simulink model "MPC_MG_raw_ver1"  (R2021b)
settings: Solver=ode23tb  StartTime=0.0  StopTime=1  RelTol=1e-3
model workspace (MAT data in the model file):
  Ts = Simulink.Parameter
  Ts.Value = 5e-06
  Ts.DataType = 'auto'
  Ts.Complexity = 'real'
  Ts.Dimensions = [1 1]
  secondary_on = Simulink.Parameter
  secondary_on.DataType = 'auto'
  secondary_on.Complexity = 'real'
  secondary_on.Dimensions = [0 0]
values from neighbouring files (symbols this model uses):
  A = zeros(4,4)    [MPC_MG_script_raw_dmpc.m]    (also in MPG_MG_July.m = [0 1 1 1; 1 0 0 0; 1 0 0 0; 1 0 0 0]; MPG_MG_freq_script.m = ones(4) - eye(4); Script.m = [0 1 1 1 ; 1 0 1 1 ; 1 1 0 1 ; 1 1 1 0])
  a12 = 0    [Four_DG_MG_PrimaryOnlyScript.m]    (also in MPC_MG_script_raw_dmpc.m; MPC_MG_secondary_script.m)
  a14 = 0    [Four_DG_MG_PrimaryOnlyScript.m]    (also in MPC_MG_script_raw_dmpc.m; MPC_MG_secondary_script.m)
  a21 = 1    [Four_DG_MG_PrimaryOnlyScript.m]    (also in MPC_MG_script_raw_dmpc.m; MPC_MG_secondary_script.m)
  a23 = 0    [Four_DG_MG_PrimaryOnlyScript.m]    (also in MPC_MG_script_raw_dmpc.m; MPC_MG_secondary_script.m)
  a32 = 1    [Four_DG_MG_PrimaryOnlyScript.m]    (also in MPC_MG_script_raw_dmpc.m; MPC_MG_secondary_script.m)
  a34 = 0    [Four_DG_MG_PrimaryOnlyScript.m]    (also in MPC_MG_script_raw_dmpc.m; MPC_MG_secondary_script.m)
  a41 = 1    [Four_DG_MG_PrimaryOnlyScript.m]    (also in MPC_MG_script_raw_dmpc.m; MPC_MG_secondary_script.m)
  a43 = 0    [Four_DG_MG_PrimaryOnlyScript.m]    (also in MPC_MG_script_raw_dmpc.m; MPC_MG_secondary_script.m)
  b1v = 1    [Four_DG_MG_PrimaryOnlyScript.m]    (also in MPC_MG_script_raw_dmpc.m; MPC_MG_secondary_script.m; MPG_MG_July.m; MPG_MG_freq_script.m)
  b1w = 1    [Four_DG_MG_PrimaryOnlyScript.m]    (also in MPC_MG_script_raw_dmpc.m; MPC_MG_secondary_script.m; MPG_MG_July.m; MPG_MG_freq_script.m)
  b2v = 0    [Four_DG_MG_PrimaryOnlyScript.m]    (also in MPC_MG_script_raw_dmpc.m; MPC_MG_secondary_script.m; MPG_MG_July.m; MPG_MG_freq_script.m)
  b2w = 0    [Four_DG_MG_PrimaryOnlyScript.m]    (also in MPC_MG_script_raw_dmpc.m; MPC_MG_secondary_script.m; MPG_MG_July.m; MPG_MG_freq_script.m)
  b3v = 0    [Four_DG_MG_PrimaryOnlyScript.m]    (also in MPC_MG_script_raw_dmpc.m; MPC_MG_secondary_script.m; MPG_MG_July.m; MPG_MG_freq_script.m)
  b3w = 0    [Four_DG_MG_PrimaryOnlyScript.m]    (also in MPC_MG_script_raw_dmpc.m; MPC_MG_secondary_script.m; MPG_MG_July.m; MPG_MG_freq_script.m)
  b4v = 0    [Four_DG_MG_PrimaryOnlyScript.m]    (also in MPC_MG_script_raw_dmpc.m; MPC_MG_secondary_script.m; MPG_MG_July.m; MPG_MG_freq_script.m)
  b4w = 0    [Four_DG_MG_PrimaryOnlyScript.m]    (also in MPC_MG_script_raw_dmpc.m; MPC_MG_secondary_script.m; MPG_MG_July.m; MPG_MG_freq_script.m)
  C_f = 50e-6    (= 5e-05)    [Four_DG_MG_PrimaryOnlyScript.m]    (also in MPC_MG_script.m; MPC_MG_script_raw_dmpc.m; MPC_MG_secondary_script.m; MPG_MG_July.m)
  cf = 60    [Four_DG_MG_PrimaryOnlyScript.m]    (also in MPC_MG_script_raw_dmpc.m = 40; MPC_MG_secondary_script.m = 40; MPG_MG_July.m = 100; MPG_MG_freq_script.m = 100)
  cv = 60    [Four_DG_MG_PrimaryOnlyScript.m]    (also in MPC_MG_script_raw_dmpc.m = 40; MPC_MG_secondary_script.m = 40; MPG_MG_July.m = 100; MPG_MG_freq_script.m = 100)
  f_c = 5000    [Four_DG_MG_PrimaryOnlyScript.m]    (also in MPC_MG_script.m = 40000; MPC_MG_script_raw_dmpc.m = 40000; MPC_MG_secondary_script.m = 40000; MPG_MG_July.m = 50000)
  kL = 1e-5    (= 1e-05)    [Four_DG_MG_PrimaryOnlyScript.m]    (also in MPC_MG_script.m = 1e-08; MPC_MG_script_raw_dmpc.m = 1e-08; MPC_MG_secondary_script.m = 1e-07; MPG_MG_July.m = 1e-07)
  L_f = 1.35e-3    (= 0.00135)    [Four_DG_MG_PrimaryOnlyScript.m]    (also in MPC_MG_script.m; MPC_MG_script_raw_dmpc.m; MPC_MG_secondary_script.m; MPG_MG_July.m)
  L_in1 = 0.35e-3    (= 0.00035)    [Four_DG_MG_PrimaryOnlyScript.m]    (also in MPC_MG_script.m; MPC_MG_script_raw_dmpc.m; MPC_MG_secondary_script.m; MPG_MG_July.m)
  L_in2 = 0.35e-3    (= 0.00035)    [Four_DG_MG_PrimaryOnlyScript.m]    (also in MPC_MG_script.m; MPC_MG_script_raw_dmpc.m; MPC_MG_secondary_script.m; MPG_MG_July.m)
  L_in3 = 0.35e-3    (= 0.00035)    [Four_DG_MG_PrimaryOnlyScript.m]    (also in MPC_MG_script.m; MPC_MG_script_raw_dmpc.m; MPC_MG_secondary_script.m; MPG_MG_July.m)
  lambda1 = [30000 50000 90000 50000]'    [MPC_MG_script_raw_dmpc.m]    (also in MPG_MG_July.m = [4 4 4 4]'; MPG_MG_freq_script.m = [3 3 3 3]'; Script.m = [1 1 1 1]')
  lambda2 = [5 6 7 6]'    [MPC_MG_script_raw_dmpc.m]    (also in MPG_MG_July.m = [0.5e-2 0.5e-2 0.5e-2 0.5e-2]'; MPG_MG_freq_script.m = [1.1 1.9 1.5 1.2]'; Script.m = [0.8e-2 0.8e-2 0.8e-2 0.8e-2]')
  lambda3 = [80000 80000 900000 80000]'    [MPC_MG_script_raw_dmpc.m]    (also in MPG_MG_July.m = [1e-3 1e-3 1e-3 1e-3]'; MPG_MG_freq_script.m = [9e-4 1.2e-2 3e-3 3e-3]'; Script.m = [1.5e-3 1.5e-3 1.5e-3 1.5e-3]')
  lambda4 = [5000 5000 5000 5000]'    [MPC_MG_script_raw_dmpc.m]
  lambda5 = [150 130 200 130]'    [MPC_MG_script_raw_dmpc.m]
  lambda6 = [5000 2000 1000 2000]'    [MPC_MG_script_raw_dmpc.m]
  LD_ref1 = 800e-6    (= 0.0008)    [Four_DG_MG_PrimaryOnlyScript.m]    (also in MPC_MG_script.m = 0.0003; MPC_MG_script_raw_dmpc.m = 0.0003; MPC_MG_secondary_script.m = 0.0001; MPG_MG_July.m = 0.0004)
  lo_co = 0.2    [Four_DG_MG_PrimaryOnlyScript.m]    (also in MPC_MG_script.m = 0.05; MPC_MG_script_raw_dmpc.m = 0.1; MPC_MG_secondary_script.m = 0.08; MPG_MG_July.m = 0.15)
  m_p1 = 9.4e-5/droopDivide    (= 9.4e-05)    [Four_DG_MG_PrimaryOnlyScript.m]    (also in MPC_MG_script.m; MPC_MG_script_raw_dmpc.m; MPC_MG_secondary_script.m; MPG_MG_July.m)
  m_p2 = 9.4e-5/droopDivide    (= 9.4e-05)    [Four_DG_MG_PrimaryOnlyScript.m]    (also in MPC_MG_script.m; MPC_MG_script_raw_dmpc.m; MPC_MG_secondary_script.m; MPG_MG_July.m)
  m_p3 = 12.5e-5/droopDivide    (= 0.000125)    [Four_DG_MG_PrimaryOnlyScript.m]    (also in MPC_MG_script.m; MPC_MG_script_raw_dmpc.m; MPC_MG_secondary_script.m; MPG_MG_July.m)
  m_p4 = 12.5e-5/droopDivide    (= 0.000125)    [Four_DG_MG_PrimaryOnlyScript.m]    (also in MPC_MG_script.m; MPC_MG_script_raw_dmpc.m; MPC_MG_secondary_script.m; MPG_MG_July.m)
  n_q1 = 1.3e-3/droopDivide2    (= 0.00013)    [Four_DG_MG_PrimaryOnlyScript.m]    (also in MPC_MG_script.m; MPC_MG_script_raw_dmpc.m; MPC_MG_secondary_script.m; MPG_MG_July.m)
  n_q2 = 1.3e-3/droopDivide2    (= 0.00013)    [Four_DG_MG_PrimaryOnlyScript.m]    (also in MPC_MG_script.m; MPC_MG_script_raw_dmpc.m; MPC_MG_secondary_script.m; MPG_MG_July.m)
  n_q3 = 1.5e-3/droopDivide2    (= 0.00015)    [Four_DG_MG_PrimaryOnlyScript.m]    (also in MPC_MG_script.m; MPC_MG_script_raw_dmpc.m; MPC_MG_secondary_script.m; MPG_MG_July.m)
  n_q4 = 1.5e-3/droopDivide2    (= 0.00015)    [Four_DG_MG_PrimaryOnlyScript.m]    (also in MPC_MG_script.m; MPC_MG_script_raw_dmpc.m; MPC_MG_secondary_script.m; MPG_MG_July.m)
  R_f = 0.1    [Four_DG_MG_PrimaryOnlyScript.m]    (also in MPC_MG_script.m; MPC_MG_script_raw_dmpc.m; MPC_MG_secondary_script.m; MPG_MG_July.m)
  R_in1 = 0.03    [Four_DG_MG_PrimaryOnlyScript.m]    (also in MPC_MG_script.m; MPC_MG_script_raw_dmpc.m; MPC_MG_secondary_script.m; MPG_MG_July.m)
  R_in2 = 0.03    [Four_DG_MG_PrimaryOnlyScript.m]    (also in MPC_MG_script.m; MPC_MG_script_raw_dmpc.m; MPC_MG_secondary_script.m; MPG_MG_July.m)
  R_in3 = 0.03    [Four_DG_MG_PrimaryOnlyScript.m]    (also in MPC_MG_script.m; MPC_MG_script_raw_dmpc.m; MPC_MG_secondary_script.m; MPG_MG_July.m)
  Smax = [45e3 45e3 37e3 37e3]'    [MPC_MG_script_raw_dmpc.m]
  Smax1 = 2400    [MPC_MG_script_raw_dmpc.m]
  Smax2 = 2400    [MPC_MG_script_raw_dmpc.m]
  Smax3 = 2400    [MPC_MG_script_raw_dmpc.m]
  Smax4 = 2400    [MPC_MG_script_raw_dmpc.m]
  time_thresh = 0.6    [Four_DG_MG_PrimaryOnlyScript.m]    (also in MPC_MG_script_raw_dmpc.m = 2; MPC_MG_secondary_script.m = 2; MPG_MG_July.m = 0.5; MPG_MG_freq_script.m = 0.5)
  Ts = 10e-6    (= 1e-05)    [Four_DG_MG_PrimaryOnlyScript.m]    (also in MPC_MG_script.m; MPC_MG_script_raw_dmpc.m; MPC_MG_secondary_script.m; MPG_MG_July.m)
  V_nom = 220*sqrt(2)    [Four_DG_MG_PrimaryOnlyScript.m]    (also in MPC_MG_script.m; MPC_MG_script_raw_dmpc.m; MPC_MG_secondary_script.m; MPG_MG_July.m)
  Vdc = 600    [Four_DG_MG_PrimaryOnlyScript.m]    (also in MPC_MG_script.m; MPC_MG_script_raw_dmpc.m; MPC_MG_secondary_script.m; MPG_MG_July.m)
  Vmax = 155    [MPC_MG_script_raw_dmpc.m]
  Vmin = 145    [MPC_MG_script_raw_dmpc.m]
  w_c_high = 2*pi*50    (= 314.159265359)    [Four_DG_MG_PrimaryOnlyScript.m]    (also in MPC_MG_script.m; MPC_MG_script_raw_dmpc.m; MPC_MG_secondary_script.m; MPG_MG_July.m)
  w_nom = 2*pi*50    (= 314.159265359)    [Four_DG_MG_PrimaryOnlyScript.m]    (also in MPC_MG_script.m; MPC_MG_script_raw_dmpc.m; MPC_MG_secondary_script.m; MPG_MG_July.m)
undefined symbols (not defined in the file or in its folder): i
libraries: spsThreePhaseSeriesRLCBranchLib x18, spsThreePhaseVIMeasurementLib x16, spsabctodq0Lib x16, eeGeneralControl x10, spsPLL3phLib x8, dspswit3 x5, powerlib x5, spsPMUPLLBasedPositiveSequenceLib x4, spsDCVoltageSourceLib x4, spsSeriesRLCBranchLib x4, spsTwoLevelConverterLib x4, spsThreePhaseSeriesRLCLoadLib x3
(part 1 of 4)
settings Model: SimulationMode=accelerator  Creator=Linh  LastModifiedBy=Linh
settings SolverCC: AlgebraicLoopSolver=TrustRegion
settings DataIOCC: ReturnWorkspaceOutputs=off
settings DebuggingCC: SFMachineParentedDataDiag=warning

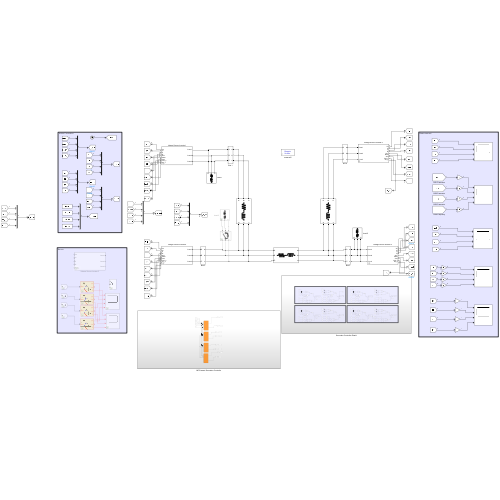
[thumbnail: Simulink's stored preview of the top-level diagram]
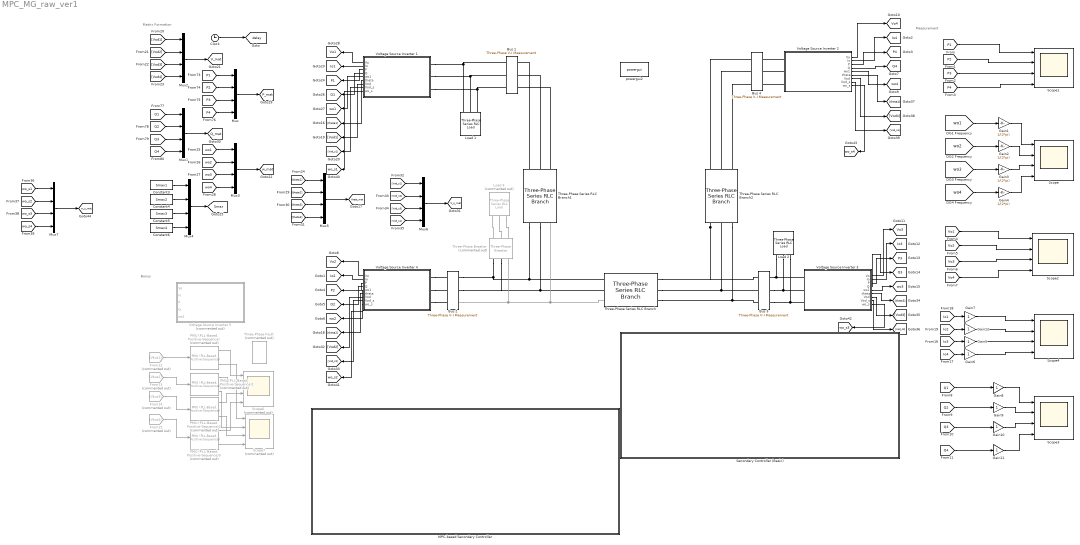
== system MPC_MG_raw_ver1 ==
  note: Bonus
  note: Matrix Formation
  note: Measurement
  Bus 1 : spsThreePhaseVIMeasurementLib/Three-Phase V-I Measurement  VoltageMeasurement=phase-to-ground  SetLabelV=on  LabelV=Vbus1  Vpu=on  VpuLL=off  CurrentMeasurement=yes  SetLabelI=on  LabelI=Ibus1  Ipu=off  Pbase=100e6  Vbase=380  OutputType=Complex  PhasorSimulation=off  PSBequivalent=0
  Bus 2 : spsThreePhaseVIMeasurementLib/Three-Phase V-I Measurement  VoltageMeasurement=phase-to-ground  SetLabelV=on  LabelV=Vbus2  Vpu=on  VpuLL=off  CurrentMeasurement=yes  SetLabelI=on  LabelI=Ibus2  Ipu=off  Pbase=100e6  Vbase=380  OutputType=Complex  PhasorSimulation=off  PSBequivalent=0
  Bus 3 : spsThreePhaseVIMeasurementLib/Three-Phase V-I Measurement  VoltageMeasurement=phase-to-ground  SetLabelV=on  LabelV=Vbus3  Vpu=on  VpuLL=off  CurrentMeasurement=yes  SetLabelI=on  LabelI=Ibus3  Ipu=off  Pbase=100e6  Vbase=380  OutputType=Complex  PhasorSimulation=off  PSBequivalent=0
  Bus 4 : spsThreePhaseVIMeasurementLib/Three-Phase V-I Measurement  VoltageMeasurement=phase-to-phase  SetLabelV=on  LabelV=Vbus4  Vpu=off  VpuLL=on  CurrentMeasurement=no  SetLabelI=off  LabelI=Ibus4  Ipu=off  Pbase=100e6  Vbase=380  OutputType=Complex  PhasorSimulation=off  PSBequivalent=0
  Clock : Clock
  Constant3 : Constant  Value=Smax1
  Constant4 : Constant  Value=Smax2
  Constant5 : Constant  Value=Smax3
  Constant6 : Constant  Value=Smax4
  From12 : From  Commented=on  GotoTag=Vbus1  TagVisibility=global
  From13 : From  Commented=on  GotoTag=Vbus2  TagVisibility=global
  From14 : From  Commented=on  GotoTag=Vbus3  TagVisibility=global
  From15 : From  Commented=on  GotoTag=Vbus4  TagVisibility=global
  Gain{1..4} (4 alike) : Gain  Gain=1/(2*pi)
  Gain{5..12} (8 alike) : Gain
  Load 1 : spsThreePhaseSeriesRLCLoadLib/Three-Phase Series RLC Load  LConnTagsString=A|B|C  Configuration=Y (grounded)  NominalVoltage=220*sqrt(3)  Vabc=[1e3 1e3 1e3]  Vabcp=[1e3 1e3 1e3]  NominalFrequency=50  UnbalancedPower=off  ActivePower=12000*3  InductivePower=12000*3  CapacitivePower=0  Pabc=[10e3 9e3 11e3]  QLabc=[100 90 110]  QCabc=[100 90 110]  Pabcp=[10e3 9e3 11e3]  QLabcp=[100 90 110]  QCabcp=[100 90 110]  Measurements=Branch voltages and currents  LoadType=constant Z
  Load 2 : spsThreePhaseSeriesRLCLoadLib/Three-Phase Series RLC Load  LConnTagsString=A|B|C  Configuration=Y (grounded)  NominalVoltage=220*sqrt(3)  Vabc=[1e3 1e3 1e3]  Vabcp=[1e3 1e3 1e3]  NominalFrequency=50  UnbalancedPower=off  ActivePower=15300*3  InductivePower=7600*3  CapacitivePower=0  Pabc=[10e3 9e3 11e3]  QLabc=[100 90 110]  QCabc=[100 90 110]  Pabcp=[10e3 9e3 11e3]  QLabcp=[100 90 110]  QCabcp=[100 90 110]  Measurements=Branch voltages and currents  LoadType=constant Z
  Load 3 : spsThreePhaseSeriesRLCLoadLib/Three-Phase Series RLC Load  Commented=on  LConnTagsString=A|B|C  Configuration=Y (grounded)  NominalVoltage=220*sqrt(3)  Vabc=[1e3 1e3 1e3]  Vabcp=[1e3 1e3 1e3]  NominalFrequency=50  UnbalancedPower=off  ActivePower=20000*3  InductivePower=12000*3  CapacitivePower=0  Pabc=[10e3 9e3 11e3]  QLabc=[100 90 110]  QCabc=[100 90 110]  Pabcp=[10e3 9e3 11e3]  QLabcp=[100 90 110]  QCabcp=[100 90 110]  Measurements=Branch voltages and currents  LoadType=constant Z
  MPC-based Secondary Controller : Subsystem
  Mux{,1..7} (8 alike) : Mux
  PMU (PLL-Based, Positive-Sequence){,1..3} (4 alike) : spsPMUPLLBasedPositiveSequenceLib/PMU (PLL-Based, Positive-Sequence)  Commented=on  nominalFrequency=50  samplingRate=64  reportingFactor=5
      settings: SourceProductBaseCode=PS
  Scope{,1..4} (5 alike) : Scope  NumInputPorts=4
  Scope6 : Scope  Commented=on  NumInputPorts=4
  Scope7 : Scope  Commented=on  NumInputPorts=4
  Secondary Controller (Basic) : Subsystem
  Three-Phase Series RLC Branch : spsThreePhaseSeriesRLCBranchLib/Three-Phase Series RLC Branch  LConnTagsString=A|B|C  RConnTagsString=A|B|C  BranchType=RL  Resistance=0.35  Inductance=1847e-6  Capacitance=1e-6  Measurements=Branch voltages and currents
  Three-Phase Series RLC Branch1 : spsThreePhaseSeriesRLCBranchLib/Three-Phase Series RLC Branch  LConnTagsString=A|B|C  RConnTagsString=A|B|C  BranchType=RL  Resistance=0.23  Inductance=318e-6  Capacitance=1e-6  Measurements=Branch voltages and currents
  Three-Phase Series RLC Branch2 : spsThreePhaseSeriesRLCBranchLib/Three-Phase Series RLC Branch  LConnTagsString=A|B|C  RConnTagsString=A|B|C  BranchType=RL  Resistance=0.23  Inductance=318e-6  Capacitance=1e-6  Measurements=Branch voltages and currents
  Three-Phase Breaker : spsThreePhaseBreakerLib/Three-Phase Breaker  Commented=on  InitialState=open  SwitchA=on  SwitchB=on  SwitchC=on  SwitchTimes="[0.5  2]"  External=off  BreakerResistance=0.01  SnubberResistance=1e6  SnubberCapacitance=inf  Measurements=None
  Three-Phase Fault : spsThreePhaseFaultLib/Three-Phase Fault  Commented=on  InitialStates=0  FaultA=on  FaultB=on  FaultC=off  GroundFault=off  SwitchTimes="[0.2  0.24]"  External=off  SwitchStatus=NaN  FaultResistance=0.001  GroundResistance=0.01  SnubberResistance=1e6  SnubberCapacitance=inf  Measurements=None
  Voltage Source Inverter 1 : Subsystem  mask{w_nom=w_nom, V_nom=V_nom, modT=1/f_c, m_p=m_p2, n_q=n_q2, LD_ref=LD_ref1, k_LD=kL, w_c_high=[1 w_c_high], R_f=R_f, L_f=L_f, C_f=C_f, R_in=R_in2, L_in=L_in2}
      mask prompts: w_nom "Nominal frequency (radian)"; V_nom "Nominal voltage"; modT "Sampling Time"; m_p "P-w gain"; n_q "Q-V gain"; LD_ref "Reference virtual impedance (H)"; k_LD "Virtual impedance Q gain"; w_c_high "High-pass filter denominator:"; R_f "Inductor resistance:"; L_f "Filter inductance"; C_f "Filter capacitance"; R_in "Resistance coupling"; L_in "Inductance coupling"
      mask TypeOptions w_nom: w_nom/Value
      mask TypeOptions V_nom: V_nom/Value
      mask TypeOptions modT:
      | Model Predictive Control
      | /Ts
      mask TypeOptions m_p: Droop for secondary control2/Gain5/Gain
      mask TypeOptions n_q: Droop for secondary control2/Gain4/Gain
      mask TypeOptions LD_ref: LD_ref/Value
      mask TypeOptions k_LD: k_LD/Gain
      mask TypeOptions w_c_high: High-Pass Filter/Denominator
      mask TypeOptions R_f:
      | Three-Phase
      | Series RLC Branch/Resistance
      mask TypeOptions L_f:
      | Three-Phase
      | Series RLC Branch/Inductance
      mask TypeOptions C_f:
      | Three-Phase
      | Series RLC Branch2/Capacitance
      mask TypeOptions R_in:
      | Three-Phase
      | Series RLC Branch1/Resistance
      mask TypeOptions L_in:
      | Three-Phase
      | Series RLC Branch1/Inductance
      mask DialogControl ParameterGroupVar Prompt: Microgrid-wide values
      mask DialogControl Container5 Prompt: Droop value
      mask DialogControl Container8 Prompt: Filter
  Voltage Source Inverter 2 : Subsystem  mask{w_nom=w_nom, V_nom=V_nom, modT=1/f_c, m_p=m_p3, n_q=n_q3, LD_ref=LD_ref1, k_LD=kL, w_c_high=[1 w_c_high], R_f=R_f, L_f=L_f, C_f=C_f, R_in=R_in3, L_in=L_in3}
      mask prompts: w_nom "Nominal frequency (radian)"; V_nom "Nominal voltage"; modT "Sampling Time"; m_p "P-w gain"; n_q "Q-V gain"; LD_ref "Reference virtual impedance (H)"; k_LD "Virtual impedance Q gain"; w_c_high "High-pass filter denominator:"; R_f "Inductor resistance:"; L_f "Filter inductance"; C_f "Filter capacitance"; R_in "Resistance coupling"; L_in "Inductance coupling"
      mask TypeOptions w_nom: w_nom/Value
      mask TypeOptions V_nom: V_nom/Value
      mask TypeOptions modT:
      | Model Predictive Control
      | /Ts
      mask TypeOptions m_p: Droop for secondary control2/Gain5/Gain
      mask TypeOptions n_q: Droop for secondary control2/Gain4/Gain
      mask TypeOptions LD_ref: LD_ref/Value
      mask TypeOptions k_LD: k_LD/Gain
      mask TypeOptions w_c_high: High-Pass Filter/Denominator
      mask TypeOptions R_f:
      | Three-Phase
      | Series RLC Branch/Resistance
      mask TypeOptions L_f:
      | Three-Phase
      | Series RLC Branch/Inductance
      mask TypeOptions C_f:
      | Three-Phase
      | Series RLC Branch2/Capacitance
      mask TypeOptions R_in:
      | Three-Phase
      | Series RLC Branch1/Resistance
      mask TypeOptions L_in:
      | Three-Phase
      | Series RLC Branch1/Inductance
      mask DialogControl ParameterGroupVar Prompt: Microgrid-wide values
      mask DialogControl Container5 Prompt: Droop value
      mask DialogControl Container8 Prompt: Filter
  Voltage Source Inverter 3 : Subsystem  mask{w_nom=w_nom, V_nom=V_nom, modT=1/f_c, m_p=m_p3, n_q=n_q3, LD_ref=LD_ref1, k_LD=kL, w_c_high=[1 w_c_high], R_f=R_f, L_f=L_f, C_f=C_f, R_in=R_in3, L_in=L_in3}
      mask prompts: w_nom "Nominal frequency (radian)"; V_nom "Nominal voltage"; modT "Sampling Time"; m_p "P-w gain"; n_q "Q-V gain"; LD_ref "Reference virtual impedance (H)"; k_LD "Virtual impedance Q gain"; w_c_high "High-pass filter denominator:"; R_f "Inductor resistance:"; L_f "Filter inductance"; C_f "Filter capacitance"; R_in "Resistance coupling"; L_in "Inductance coupling"
      mask TypeOptions w_nom: w_nom/Value
      mask TypeOptions V_nom: V_nom/Value
      mask TypeOptions modT:
      | Model Predictive Control
      | /Ts
      mask TypeOptions m_p: Droop for secondary control2/Gain5/Gain
      mask TypeOptions n_q: Droop for secondary control2/Gain4/Gain
      mask TypeOptions LD_ref: LD_ref/Value
      mask TypeOptions k_LD: k_LD/Gain
      mask TypeOptions w_c_high: High-Pass Filter/Denominator
      mask TypeOptions R_f:
      | Three-Phase
      | Series RLC Branch/Resistance
      mask TypeOptions L_f:
      | Three-Phase
      | Series RLC Branch/Inductance
      mask TypeOptions C_f:
      | Three-Phase
      | Series RLC Branch2/Capacitance
      mask TypeOptions R_in:
      | Three-Phase
      | Series RLC Branch1/Resistance
      mask TypeOptions L_in:
      | Three-Phase
      | Series RLC Branch1/Inductance
      mask DialogControl ParameterGroupVar Prompt: Microgrid-wide values
      mask DialogControl Container5 Prompt: Droop value
      mask DialogControl Container8 Prompt: Filter
  Voltage Source Inverter 4 : Subsystem  mask{w_nom=w_nom, V_nom=V_nom, modT=1/f_c, m_p=m_p2, n_q=n_q2, LD_ref=LD_ref1, k_LD=kL, w_c_high=[1 w_c_high], R_f=R_f, L_f=L_f, C_f=C_f, R_in=R_in2, L_in=L_in2}
      mask prompts: w_nom "Nominal frequency (radian)"; V_nom "Nominal voltage"; modT "Sampling Time"; m_p "P-w gain"; n_q "Q-V gain"; LD_ref "Reference virtual impedance (H)"; k_LD "Virtual impedance Q gain"; w_c_high "High-pass filter denominator:"; R_f "Inductor resistance:"; L_f "Filter inductance"; C_f "Filter capacitance"; R_in "Resistance coupling"; L_in "Inductance coupling"
      mask TypeOptions w_nom: w_nom/Value
      mask TypeOptions V_nom: V_nom/Value
      mask TypeOptions modT:
      | Model Predictive Control
      | /Ts
      mask TypeOptions m_p: Droop for secondary control2/Gain5/Gain
      mask TypeOptions n_q: Droop for secondary control2/Gain4/Gain
      mask TypeOptions LD_ref: LD_ref/Value
      mask TypeOptions k_LD: k_LD/Gain
      mask TypeOptions w_c_high: High-Pass Filter/Denominator
      mask TypeOptions R_f:
      | Three-Phase
      | Series RLC Branch/Resistance
      mask TypeOptions L_f:
      | Three-Phase
      | Series RLC Branch/Inductance
      mask TypeOptions C_f:
      | Three-Phase
      | Series RLC Branch2/Capacitance
      mask TypeOptions R_in:
      | Three-Phase
      | Series RLC Branch1/Resistance
      mask TypeOptions L_in:
      | Three-Phase
      | Series RLC Branch1/Inductance
      mask DialogControl ParameterGroupVar Prompt: Microgrid-wide values
      mask DialogControl Container5 Prompt: Droop value
      mask DialogControl Container8 Prompt: Filter
  Voltage Source Inverter 5 : Subsystem  Commented=on  mask{w_nom=w_nom, V_nom=V_nom, modT=1/f_c, m_p=m_p1, n_q=n_q1, LD_ref=LD_ref1, k_LD=kL, w_c_high=[1 w_c_high], R_f=R_f, L_f=L_f, C_f=C_f, R_in=R_in1, L_in=L_in1}
      mask prompts: w_nom "Nominal frequency (radian)"; V_nom "Nominal voltage"; modT "Sampling Time"; m_p "P-w gain"; n_q "Q-V gain"; LD_ref "Reference virtual impedance (H)"; k_LD "Virtual impedance Q gain"; w_c_high "High-pass filter denominator:"; R_f "Inductor resistance:"; L_f "Filter inductance"; C_f "Filter capacitance"; R_in "Resistance coupling"; L_in "Inductance coupling"
      mask TypeOptions w_nom: w_nom/Value
      mask TypeOptions V_nom: V_nom/Value
      mask TypeOptions modT:
      | Model Predictive Control
      | /Ts
      mask TypeOptions m_p: Droop for secondary control2/Gain5/Gain
      mask TypeOptions n_q: Droop for secondary control2/Gain4/Gain
      mask TypeOptions LD_ref: LD_ref/Value
      mask TypeOptions k_LD: k_LD/Gain
      mask TypeOptions w_c_high: High-Pass Filter/Denominator
      mask TypeOptions R_f:
      | Three-Phase
      | Series RLC Branch/Resistance
      mask TypeOptions L_f:
      | Three-Phase
      | Series RLC Branch/Inductance
      mask TypeOptions C_f:
      | Three-Phase
      | Series RLC Branch2/Capacitance
      mask TypeOptions R_in:
      | Three-Phase
      | Series RLC Branch1/Resistance
      mask TypeOptions L_in:
      | Three-Phase
      | Series RLC Branch1/Inductance
      mask DialogControl ParameterGroupVar Prompt: Microgrid-wide values
      mask DialogControl Container5 Prompt: Droop value
      mask DialogControl Container8 Prompt: Filter
  powergui2 : spspowerguiLib/powergui  Priority=1  SimulationMode=Discrete  SampleTime=Ts  frequency=60  Iterations=50  frequencyindice=0  Pbase=100e6  ErrMax=1e-4  UnitsV=kV  UnitsW=MW  buscounter=0  FunctionMessages=off  echomessages=off  EnableUseOfTLC=off  CurrentSourceSwitches=off  DisableSnubberDevices=off  DisableRonSwitches=off  DisableVfSwitches=off  DisplayEquations=off  AutomaticDiscreteSolvers=off  SolverType=Tustin/Backward Euler (TBE)  Interpol=off  ExternalGateDelay=off  methode=off  Ts=100  x0status=blocks  SPID=on  SwTol=0  HookPort=off  NonlinearTolerance=1e-4  nMaxIteration=100  ContinueOnMaxIteration=off  RestoreLinks=warning  ResistiveCurrentMeasurement=off  Frange=[0:2:500]  Ylog=off  Xlog=on  ShowGrid=off  save=off  variable=ZData  structure=ScopeData3  ZoomFFT=off  StartTime=0.5  cycles=1  DisplayStyle=1  fundamental=50  FreqAxis=off  MaxFrequency=1000  frequencyindicesteady=1  RmsSteady=1  display=off
  tag scope: Io1=global, Io2=global, Io3=global, Io4=global, P1=global, P2=global, P3=global, P4=global, P_mat=global, Q1=global, Q2=global, Q3=global, Q4=global, Q_mat=global, Smax=global, V_mat=global, V_s_mat=global, Vo1=global, Vo2=global, Vo3=global, Vo4=global, delay=global, theta_mat=global, w_mat=global, w_s_mat=global, wo1=global, wo2=global, wo3=global, wo4=global, wo_s1=global, wo_s2=global, wo_s3=global, wo_s4=global
  wires:
  "PMU (PLL-Based, Positive-Sequence)1"/3 -> Scope7/2
  From12/1 -> "PMU (PLL-Based, Positive-Sequence)"/1
  Gain8/1 -> Scope3/1
  Gain11/1 -> Scope3/4
  [Q4] -> Gain11/1
  [Q1] -> Gain8/1
  [wo3] -> Gain3/1
  "PMU (PLL-Based, Positive-Sequence)3"/1 -> Scope6/4
  Gain2/1 -> Scope/2
  Gain4/1 -> Scope/4
  "PMU (PLL-Based, Positive-Sequence)2"/3 -> Scope7/3
  [wo1] -> Gain1/1
  "PMU (PLL-Based, Positive-Sequence)2"/1 -> Scope6/3
  From14/1 -> "PMU (PLL-Based, Positive-Sequence)2"/1
  [P1] -> Scope1/1
  "PMU (PLL-Based, Positive-Sequence)3"/3 -> Scope7/4
  "PMU (PLL-Based, Positive-Sequence)"/1 -> Scope6/1
  "PMU (PLL-Based, Positive-Sequence)"/3 -> Scope7/1
  "PMU (PLL-Based, Positive-Sequence)1"/1 -> Scope6/2
  From13/1 -> "PMU (PLL-Based, Positive-Sequence)1"/1
  [Vo4] -> Scope2/4
  [P3] -> Scope1/3
  [Q2] -> Gain9/1
  Gain9/1 -> Scope3/2
  [P2] -> Scope1/2
  Gain3/1 -> Scope/3
  [Vo2] -> Scope2/2
  [Vo3] -> Scope2/3
  [Vo1] -> Scope2/1
  [wo2] -> Gain2/1
  [Q3] -> Gain10/1
  Gain1/1 -> Scope/1
  [P4] -> Scope1/4
  Gain10/1 -> Scope3/3
  From15/1 -> "PMU (PLL-Based, Positive-Sequence)3"/1
  [wo4] -> Gain4/1
  [Io3] -> Gain5/1
  [Io1] -> Gain7/1
  [Io2] -> Gain12/1
  Gain6/1 -> Scope4/4
  [Io4] -> Gain6/1
  Gain5/1 -> Scope4/3
  Gain7/1 -> Scope4/1
  Gain12/1 -> Scope4/2
  Clock/1 -> [delay]
  [P1] -> Mux/1
  [P2] -> Mux/2
  [P3] -> Mux/3
  [P4] -> Mux/4
  Mux/1 -> [P_mat]
  [Q3] -> Mux1/3
  [Q4] -> Mux1/4
  [Q1] -> Mux1/1
  Mux1/1 -> [Q_mat]
  [Q2] -> Mux1/2
  [Vod3] -> Mux2/3
  [Vod4] -> Mux2/4
  [Vod1] -> Mux2/1
  Mux2/1 -> [V_mat]
  [Vod2] -> Mux2/2
  [wo3] -> Mux3/3
  [wo4] -> Mux3/4
  [wo1] -> Mux3/1
  Mux3/1 -> [w_mat]
  [wo2] -> Mux3/2
  Constant3/1 -> Mux4/1
  Constant4/1 -> Mux4/2
  Constant5/1 -> Mux4/3
  Constant6/1 -> Mux4/4
  Mux4/1 -> [Smax]
  Voltage Source Inverter 1/5(wo1) -> [wo1]
  Voltage Source Inverter 1/1(Vo) -> [Vo1]
  Voltage Source Inverter 1/2(Io) -> [Io1]
  Voltage Source Inverter 1/3(P) -> [P1]
  Voltage Source Inverter 1/4(Q) -> [Q1]
  Voltage Source Inverter 2/1(Vo) -> [Vo4]
  Voltage Source Inverter 2/2(Io) -> [Io4]
  Voltage Source Inverter 2/4(Q) -> [Q4]
  Voltage Source Inverter 2/3(P) -> [P4]
  Voltage Source Inverter 2/5(wo1) -> [wo4]
  Voltage Source Inverter 3/5(wo1) -> [wo3]
  Voltage Source Inverter 3/4(Q) -> [Q3]
  Voltage Source Inverter 3/1(Vo) -> [Vo3]
  Voltage Source Inverter 3/3(P) -> [P3]
  Voltage Source Inverter 3/2(Io) -> [Io3]
  Voltage Source Inverter 1/6(theta) -> [theta1]
  [theta1] -> Mux5/1
  [theta3] -> Mux5/3
  [theta2] -> Mux5/2
  Mux5/1 -> [theta_mat]
  [theta4] -> Mux5/4
  Voltage Source Inverter 1/7(Vod) -> [Vod1]
  Voltage Source Inverter 1/8(Vod_s) -> [Vod_s1]
  [Vod_s2] -> Mux6/2
  [Vod_s3] -> Mux6/3
  [Vod_s1] -> Mux6/1
  Mux6/1 -> [V_s_mat]
  [Vod_s4] -> Mux6/4
  Voltage Source Inverter 4/1(Vo) -> [Vo2]
  Voltage Source Inverter 4/2(Io) -> [Io2]
  Voltage Source Inverter 4/3(P) -> [P2]
  Voltage Source Inverter 4/4(Q) -> [Q2]
  Voltage Source Inverter 4/5(wo1) -> [wo2]
  Voltage Source Inverter 4/6(theta) -> [theta2]
  Voltage Source Inverter 4/7(Vod) -> [Vod2]
  Voltage Source Inverter 4/8(Vod_s) -> [Vod_s2]
  Voltage Source Inverter 3/6(theta) -> [theta3]
  Voltage Source Inverter 3/7(Vod) -> [Vod3]
  Voltage Source Inverter 3/8(Vod_s) -> [Vod_s3]
  Voltage Source Inverter 2/6(theta) -> [theta4]
  Voltage Source Inverter 2/7(Vod) -> [Vod4]
  Voltage Source Inverter 2/8(Vod_s) -> [Vod_s4]
  Voltage Source Inverter 1/9(wo_s) -> [wo_s1]
  Voltage Source Inverter 4/9(wo_s) -> [wo_s2]
  Voltage Source Inverter 3/9(wo_s) -> [wo_s3]
  Voltage Source Inverter 2/9(wo_s) -> [wo_s4]
  [wo_s3] -> Mux7/3
  [wo_s2] -> Mux7/2
  [wo_s4] -> Mux7/4
  Mux7/1 -> [w_s_mat]
  [wo_s1] -> Mux7/1
  connections:
  Voltage Source Inverter 4/LConn1 -- Bus 2/LConn1
  Voltage Source Inverter 4/LConn2 -- Bus 2/LConn2
  Voltage Source Inverter 4/LConn3 -- Bus 2/LConn3
  Three-Phase Series RLC Branch1/RConn2 -- Three-Phase Series RLC Branch/LConn2 -- Three-Phase Breaker/LConn2 -- Bus 2/RConn2
  Bus 3/LConn2 -- Three-Phase Series RLC Branch/RConn2 -- Three-Phase Series RLC Branch2/RConn2
  Bus 2/RConn1 -- Three-Phase Series RLC Branch/LConn1 -- Three-Phase Series RLC Branch1/RConn1 -- Three-Phase Breaker/LConn1
  Three-Phase Breaker/LConn3 -- Three-Phase Series RLC Branch/LConn3 -- Three-Phase Series RLC Branch1/RConn3 -- Bus 2/RConn3
  Load 2/LConn2 -- Voltage Source Inverter 3/LConn2 -- Bus 3/RConn2
  Bus 3/LConn3 -- Three-Phase Series RLC Branch/RConn3 -- Three-Phase Series RLC Branch2/RConn3
  Load 2/LConn1 -- Voltage Source Inverter 3/LConn1 -- Bus 3/RConn1
  Three-Phase Series RLC Branch2/RConn1 -- Three-Phase Series RLC Branch/RConn1 -- Bus 3/LConn1
  Load 2/LConn3 -- Voltage Source Inverter 3/LConn3 -- Bus 3/RConn3
  Three-Phase Series RLC Branch1/LConn2 -- Bus 1/RConn2
  Load 3/LConn3 -- Three-Phase Breaker/RConn3
  Three-Phase Series RLC Branch2/LConn1 -- Bus 4/LConn1
  Three-Phase Breaker/RConn1 -- Load 3/LConn1
  Three-Phase Series RLC Branch1/LConn1 -- Bus 1/RConn1
  Three-Phase Series RLC Branch2/LConn3 -- Bus 4/LConn3
  Three-Phase Series RLC Branch2/LConn2 -- Bus 4/LConn2
  Three-Phase Series RLC Branch1/LConn3 -- Bus 1/RConn3
  Load 3/LConn2 -- Three-Phase Breaker/RConn2
  Voltage Source Inverter 2/LConn1 -- Bus 4/RConn1
  Voltage Source Inverter 2/LConn2 -- Bus 4/RConn2
  Voltage Source Inverter 2/LConn3 -- Bus 4/RConn3
  Bus 1/LConn1 -- Voltage Source Inverter 1/LConn1 -- Load 1/LConn1
  Bus 1/LConn2 -- Voltage Source Inverter 1/LConn2 -- Load 1/LConn2
  Bus 1/LConn3 -- Voltage Source Inverter 1/LConn3 -- Load 1/LConn3

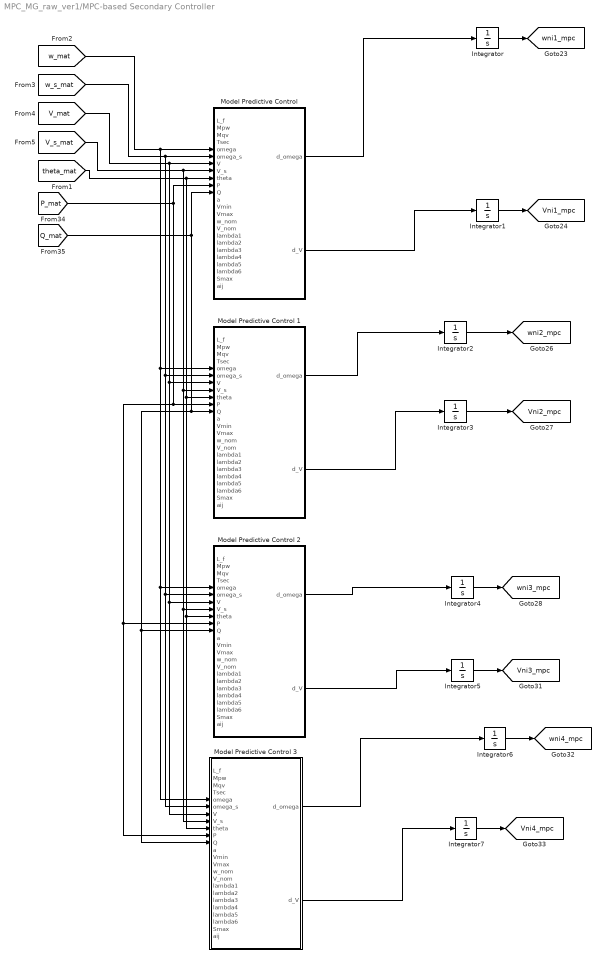
== system MPC_MG_raw_ver1/MPC-based Secondary Controller ==
  Integrator{,1..7} (8 alike) : Integrator
  "Model Predictive Control " : MATLAB Function  mask{lambda1=lambda1, lambda2=lambda2, lambda3=lambda3, lambda4=lambda4, lambda5=lambda5, lambda6=lambda6, Vmin=Vmin, Vmax=Vmax, aij=A, a=1, Smax=Smax, w_nom=w_nom, V_nom=V_nom, Mpw=1, Mqv=1, L_f=L_f, Tsec=0.1}
      mask prompts: lambda1 "Weight factor 1"; lambda2 "Weight factor 2"; lambda3 "Weight factor 3"; lambda4 "Weight factor 4"; lambda5 "Weight factor 5"; lambda6 "Weight factor 6"; aij "Adjacency matrix"; a "Inverter index"; Smax "Max total power"; w_nom "Nominal frequency"; V_nom "Nominal voltage"
  Model Predictive Control 1 : MATLAB Function  mask{lambda1=lambda1, lambda2=lambda2, lambda3=lambda3, lambda4=lambda4, lambda5=lambda5, lambda6=lambda6, Vmin=Vmin, Vmax=Vmax, aij=A, a=2, Smax=Smax, w_nom=w_nom, V_nom=V_nom, Mpw=1, Mqv=1, L_f=L_f, Tsec=0.1}
      mask prompts: lambda1 "Weight factor 1"; lambda2 "Weight factor 2"; lambda3 "Weight factor 3"; lambda4 "Weight factor 4"; lambda5 "Weight factor 5"; lambda6 "Weight factor 6"; aij "Adjacency matrix"; a "Inverter index"; Smax "Max total power"; w_nom "Nominal frequency"; V_nom "Nominal voltage"
  Model Predictive Control 2 : MATLAB Function  mask{lambda1=lambda1, lambda2=lambda2, lambda3=lambda3, lambda4=lambda4, lambda5=lambda5, lambda6=lambda6, Vmin=Vmin, Vmax=Vmax, aij=A, a=3, Smax=Smax, w_nom=w_nom, V_nom=V_nom, Mpw=1, Mqv=1, L_f=L_f, Tsec=0.1}
      mask prompts: lambda1 "Weight factor 1"; lambda2 "Weight factor 2"; lambda3 "Weight factor 3"; lambda4 "Weight factor 4"; lambda5 "Weight factor 5"; lambda6 "Weight factor 6"; aij "Adjacency matrix"; a "Inverter index"; Smax "Max total power"; w_nom "Nominal frequency"; V_nom "Nominal voltage"
  Model Predictive Control 3 : MATLAB Function  mask{lambda1=lambda1, lambda2=lambda2, lambda3=lambda3, lambda4=lambda4, lambda5=lambda5, lambda6=lambda6, Vmin=Vmin, Vmax=Vmax, aij=A, a=4, Smax=Smax, w_nom=w_nom, V_nom=V_nom, Mpw=1, Mqv=1, L_f=L_f, Tsec=0.1}
      mask prompts: lambda1 "Weight factor 1"; lambda2 "Weight factor 2"; lambda3 "Weight factor 3"; lambda4 "Weight factor 4"; lambda5 "Weight factor 5"; lambda6 "Weight factor 6"; aij "Adjacency matrix"; a "Inverter index"; Smax "Max total power"; w_nom "Nominal frequency"; V_nom "Nominal voltage"
  tag scope: Vni1_mpc=global, Vni2_mpc=global, Vni3_mpc=global, Vni4_mpc=global, wni1_mpc=global, wni2_mpc=global, wni3_mpc=global, wni4_mpc=global
  wires:
  Integrator4/1 -> [wni3_mpc]
  Integrator/1 -> [wni1_mpc]
  Integrator1/1 -> [Vni1_mpc]
  Integrator3/1 -> [Vni2_mpc]
  "Model Predictive Control "/2(d_V) -> Integrator1/1
  Integrator2/1 -> [wni2_mpc]
  Integrator5/1 -> [Vni3_mpc]
  Integrator7/1 -> [Vni4_mpc]
  Integrator6/1 -> [wni4_mpc]
  "Model Predictive Control "/1(d_omega) -> Integrator/1
  [Q_mat] -> Model Predictive Control 1/11(Q), Model Predictive Control 3/11(Q), Model Predictive Control 2/11(Q), "Model Predictive Control "/11(Q)
  [P_mat] -> Model Predictive Control 1/10(P), Model Predictive Control 3/10(P), Model Predictive Control 2/10(P), "Model Predictive Control "/10(P)
  Model Predictive Control 1/2(d_V) -> Integrator3/1
  Model Predictive Control 1/1(d_omega) -> Integrator2/1
  Model Predictive Control 2/1(d_omega) -> Integrator4/1
  Model Predictive Control 2/2(d_V) -> Integrator5/1
  Model Predictive Control 3/1(d_omega) -> Integrator6/1
  Model Predictive Control 3/2(d_V) -> Integrator7/1
  [theta_mat] -> Model Predictive Control 3/9(theta), Model Predictive Control 2/9(theta), Model Predictive Control 1/9(theta), "Model Predictive Control "/9(theta)
  [w_mat] -> Model Predictive Control 3/5(omega), Model Predictive Control 2/5(omega), Model Predictive Control 1/5(omega), "Model Predictive Control "/5(omega)
  [w_s_mat] -> Model Predictive Control 3/6(omega_s), Model Predictive Control 2/6(omega_s), Model Predictive Control 1/6(omega_s), "Model Predictive Control "/6(omega_s)
  [V_mat] -> Model Predictive Control 3/7(V), Model Predictive Control 2/7(V), Model Predictive Control 1/7(V), "Model Predictive Control "/7(V)
  [V_s_mat] -> Model Predictive Control 3/8(V_s), Model Predictive Control 2/8(V_s), Model Predictive Control 1/8(V_s), "Model Predictive Control "/8(V_s)

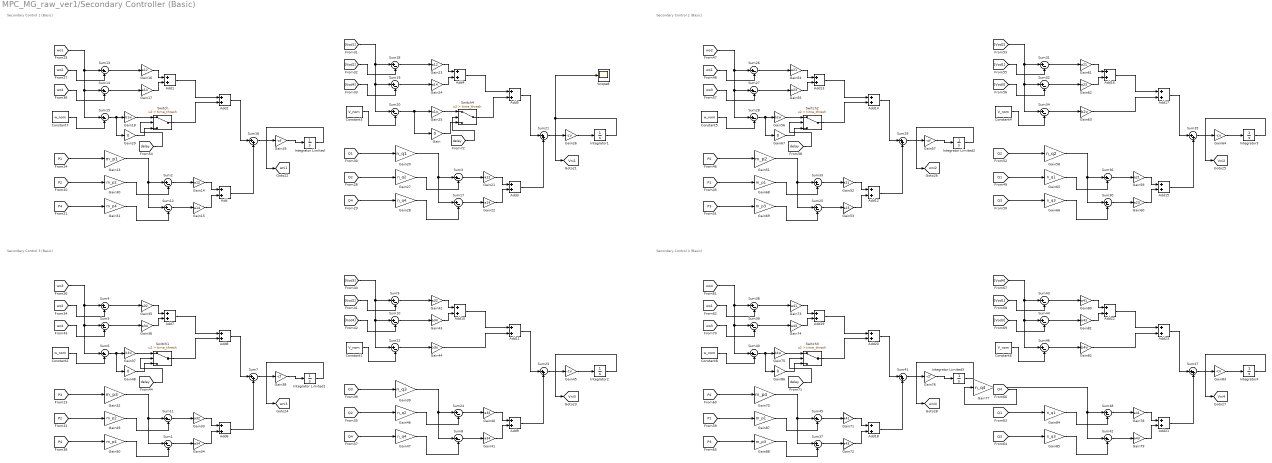
== system MPC_MG_raw_ver1/Secondary Controller (Basic) ==
  note: Secondary Control 1 (Basic)
  note: Secondary Control 3 (Basic)
  note: Secondary Control 2 (Basic)
  note: Secondary Control 4 (Basic)
  Add{,1..23} (24 alike) : Sum
  Constant{1,3..4,6} (4 alike) : Constant  Value=V_nom
  Constant{2,5,7..8} (4 alike) : Constant  Value=w_nom
  Gain{,29,48,67,86} (5 alike) : Gain  Gain=0
  Gain13 : Gain  Gain=m_p1
  Gain{14,16,21,23} (4 alike) : Gain  Gain=a12
  Gain{15,17,22,24} (4 alike) : Gain  Gain=a14
  Gain18 : Gain  Gain=b1w
  Gain{19,38,57,76} (4 alike) : Gain  Gain=-cf
  Gain20 : Gain  Gain=n_q1
  Gain25 : Gain  Gain=b1v
  Gain{26,45,64,83} (4 alike) : Gain  Gain=-cv
  Gain27 : Gain  Gain=n_q2
  Gain28 : Gain  Gain=n_q4
  Gain30 : Gain  Gain=m_p2
  Gain31 : Gain  Gain=m_p4
  Gain32 : Gain  Gain=m_p3
  Gain{33,35,40,42} (4 alike) : Gain  Gain=a32
  Gain{34,36,41,43} (4 alike) : Gain  Gain=a34
  Gain37 : Gain  Gain=b3w
  Gain39 : Gain  Gain=n_q3
  Gain44 : Gain  Gain=b3v
  Gain46 : Gain  Gain=n_q2
  Gain47 : Gain  Gain=n_q4
  Gain49 : Gain  Gain=m_p2
  Gain50 : Gain  Gain=m_p4
  Gain51 : Gain  Gain=m_p2
  Gain{52,54,59,61} (4 alike) : Gain  Gain=a21
  Gain{53,55,60,62} (4 alike) : Gain  Gain=a23
  Gain56 : Gain  Gain=b2w
  Gain58 : Gain  Gain=n_q2
  Gain63 : Gain  Gain=b2v
  Gain65 : Gain  Gain=n_q1
  Gain66 : Gain  Gain=n_q3
  Gain68 : Gain  Gain=m_p1
  Gain69 : Gain  Gain=m_p3
  Gain70 : Gain  Gain=m_p4
  Gain{71,73,78,80} (4 alike) : Gain  Gain=a41
  Gain{72,74,79,81} (4 alike) : Gain  Gain=a43
  Gain75 : Gain  Gain=b4w
  Gain77 : Gain  Gain=n_q4
  Gain82 : Gain  Gain=b4v
  Gain84 : Gain  Gain=n_q1
  Gain85 : Gain  Gain=n_q3
  Gain87 : Gain  Gain=m_p1
  Gain88 : Gain  Gain=m_p3
  Integrator Limited{,1..3} (4 alike) : Integrator  InitialCondition=50*2*pi  UpperSaturationLimit=51*2*pi  LowerSaturationLimit=50*2*pi
  Integrator{1..4} (4 alike) : Integrator  InitialCondition=311  UpperSaturationLimit=373.35  LowerSaturationLimit=248.90
  Scope8 : Scope
  Sum{1..6,8..15,17..20,22,24..28,30..34,36..40,42..46,48} (40 alike) : Sum  Inputs=|+-
  Sum{7,16,21,23,29,35,41,47} (8 alike) : Sum  Inputs=|++
  Switch{,1..4} (5 alike) : Switch  Criteria=u2 > Threshold  Threshold=time_thresh
  tag scope: Vni1=global, Vni2=global, Vni3=global, Vni4=global, wni1=global, wni2=global, wni3=global, wni4=global
  wires:
  Gain16/1 -> Add1/1
  Gain28/1 -> Sum17/2
  Gain48/1 -> Switch1/3
  [P2] -> Gain30/1
  [wo1] -> Sum13/1, Sum14/1, Sum15/1
  Integrator1/1 -> Scope8/1, [Vni1]
  Gain42/1 -> Add10/1
  [Vod1] -> Sum31/2
  Add7/1 -> Add8/1
  Sum47/1 -> Gain83/1
  Gain22/1 -> Add3/2
  Sum16/1 -> Gain19/1
  Gain18/1 -> Switch/1
  [P3] -> Gain69/1
  [Vod4] -> Sum19/2
  Sum2/1 -> Gain14/1
  [delay] -> Switch/2
  Add4/1 -> Add5/1
  [Vod4] -> Sum43/1, Sum44/1, Sum46/1
  Gain24/1 -> Add4/2
  Sum15/1 -> Gain18/1, Gain29/1
  Add13/1 -> Add14/1
  [P4] -> Gain31/1
  Sum10/1 -> Gain43/1
  Sum48/1 -> Gain78/1
  Sum17/1 -> Gain22/1
  Sum20/1 -> Gain/1, Gain25/1
  Gain13/1 -> Sum2/1, Sum12/1
  Add/1 -> Sum16/2
  Gain85/1 -> Sum42/2
  Gain50/1 -> Sum1/2
  Sum3/1 -> Gain21/1
  [wo3] -> Sum4/1, Sum5/1, Sum6/1
  Sum19/1 -> Gain24/1
  Integrator2/1 -> [Vni3]
  Gain/1 -> Switch4/3
  Sum35/1 -> Gain64/1
  Add2/1 -> Sum16/1
  Gain34/1 -> Add6/2
  Sum37/1 -> Gain72/1
  Gain14/1 -> Add/1
  Gain49/1 -> Sum11/2
  Gain20/1 -> Sum3/1, Sum17/1
  Sum11/1 -> Gain33/1
  Gain74/1 -> Add19/2
  [P1] -> Gain87/1
  Gain37/1 -> Switch1/1
  [P2] -> Gain49/1
  Sum13/1 -> Gain16/1
  Gain47/1 -> Sum8/2
  [Vod2] -> Sum18/2
  Sum9/1 -> Gain42/1
  Integrator Limited/1 -> [wni1]
  [Vod1] -> Sum18/1, Sum19/1, Sum20/1
  [wo2] -> Sum13/2
  Constant2/1 -> Sum6/2
  Gain36/1 -> Add7/2
  Gain21/1 -> Add3/1
  Sum4/1 -> Gain35/1
  [Q2] -> Gain27/1
  Gain59/1 -> Add15/1
  Add5/1 -> Sum21/1
  [wo4] -> Sum14/2
  Gain26/1 -> Integrator1/1
  Gain27/1 -> Sum3/2
  Sum21/1 -> Gain26/1
  Gain23/1 -> Add4/1
  Sum41/1 -> Gain76/1
  [Vod4] -> Sum10/2
  Gain17/1 -> Add1/2
  Sum23/1 -> Gain45/1
  [wo1] -> Sum38/2
  Add17/1 -> Sum35/1
  Gain45/1 -> Integrator2/1
  Constant1/1 -> Sum22/2
  Gain41/1 -> Add9/2
  Gain19/1 -> Integrator Limited/1
  Sum27/1 -> Gain55/1
  Gain38/1 -> Integrator Limited1/1
  Sum7/1 -> Gain38/1
  Gain39/1 -> Sum24/1, Sum8/1
  Sum30/1 -> Gain60/1
  Gain40/1 -> Add9/1
  Sum5/1 -> Gain36/1
  [Q4] -> Gain47/1
  Gain76/1 -> Integrator Limited3/1
  [wo2] -> Sum4/2
  Gain15/1 -> Add/2
  Gain30/1 -> Sum2/2
  Gain33/1 -> Add6/1
  [P4] -> Gain50/1
  [wo4] -> Sum5/2
  Gain44/1 -> Add11/2
  [Q2] -> Gain46/1
  [Q3] -> Gain39/1
  Sum8/1 -> Gain41/1
  Gain43/1 -> Add10/2
  [Vod3] -> Sum9/1, Sum10/1, Sum22/1
  Gain32/1 -> Sum11/1, Sum1/1
  Sum42/1 -> Gain79/1
  [Q3] -> Gain85/1
  Gain29/1 -> Switch/3
  Gain35/1 -> Add7/1
  Add6/1 -> Sum7/2
  Constant5/1 -> Sum28/2
  Gain46/1 -> Sum24/2
  Gain77/1 -> Sum48/1, Sum42/1
  Sum26/1 -> Gain54/1
  Gain67/1 -> Switch2/3
  Add11/1 -> Sum23/1
  [P1] -> Gain13/1
  [Vod3] -> Sum32/2
  Integrator3/1 -> [Vni2]
  Sum31/1 -> Gain61/1
  Gain82/1 -> Add23/2
  [delay] -> Switch1/2
  Gain88/1 -> Sum37/2
  Add14/1 -> Sum29/1
  Add1/1 -> Add2/1
  [P1] -> Gain68/1
  Add12/1 -> Sum29/2
  Integrator Limited1/1 -> [wni3]
  Add8/1 -> Sum7/1
  Gain66/1 -> Sum30/2
  Gain87/1 -> Sum45/2
  Gain61/1 -> Add16/1
  Integrator Limited2/1 -> [wni2]
  Gain60/1 -> Add15/2
  Sum18/1 -> Gain23/1
  Constant3/1 -> Sum20/2
  Sum22/1 -> Gain44/1
  Constant4/1 -> Sum34/2
  [Q4] -> Gain28/1
  Gain62/1 -> Add16/2
  Integrator Limited3/1 -> [wni4]
  [Q1] -> Gain84/1
  [Q1] -> Gain20/1
  Gain64/1 -> Integrator3/1
  Sum34/1 -> Gain63/1
  Gain53/1 -> Add12/2
  Gain75/1 -> Switch3/1
  [Vod2] -> Sum31/1, Sum32/1, Sum34/1
  Constant7/1 -> Sum15/2
  Gain57/1 -> Integrator Limited2/1
  Gain54/1 -> Add13/1
  [Q1] -> Gain65/1
  [wo3] -> Sum27/2
  [P3] -> Gain32/1
  [Q3] -> Gain66/1
  Gain52/1 -> Add12/1
  Add15/1 -> Sum35/2
  Sum25/1 -> Gain53/1
  Sum38/1 -> Gain73/1
  Sum45/1 -> Gain71/1
  Add21/1 -> Sum47/2
  [Vod3] -> Sum44/2
  Gain55/1 -> Add13/2
  Add10/1 -> Add11/1
  [wo1] -> Sum26/2
  [P3] -> Gain88/1
  Gain69/1 -> Sum25/2
  [Q2] -> Gain58/1
  Switch3/1 -> Add20/2
  Sum28/1 -> Gain56/1, Gain67/1
  Gain58/1 -> Sum36/1, Sum30/1
  [delay] -> Switch2/2
  Gain81/1 -> Add22/2
  Gain51/1 -> Sum33/1, Sum25/1
  [Vod1] -> Sum43/2
  Add19/1 -> Add20/1
  Gain56/1 -> Switch2/1
  Sum36/1 -> Gain59/1
  [wo4] -> Sum38/1, Sum39/1, Sum40/1
  Gain79/1 -> Add21/2
  Sum33/1 -> Gain52/1
  Sum46/1 -> Gain82/1
  Add3/1 -> Sum21/2
  [wo3] -> Sum39/2
  Add16/1 -> Add17/1
  Integrator4/1 -> [Vni4]
  Sum44/1 -> Gain81/1
  Gain84/1 -> Sum48/2
  Sum14/1 -> Gain17/1
  Switch2/1 -> Add14/2
  Gain86/1 -> Switch3/3
  Gain80/1 -> Add22/1
  Switch1/1 -> Add8/2
  [P2] -> Gain51/1
  Add23/1 -> Sum47/1
  Gain72/1 -> Add18/2
  [delay] -> Switch4/2
  Constant6/1 -> Sum46/2
  Gain83/1 -> Integrator4/1
  Gain68/1 -> Sum33/2
  Sum24/1 -> Gain40/1
  Gain31/1 -> Sum12/2
  Sum6/1 -> Gain37/1, Gain48/1
  Sum1/1 -> Gain34/1
  Sum32/1 -> Gain62/1
  Sum40/1 -> Gain75/1, Gain86/1
  Sum43/1 -> Gain80/1
  Sum29/1 -> Gain57/1
  Sum39/1 -> Gain74/1
  Gain71/1 -> Add18/1
  Sum12/1 -> Gain15/1
  [P4] -> Gain70/1
  [delay] -> Switch3/2
  Gain65/1 -> Sum36/2
  Gain63/1 -> Add17/2
  Gain70/1 -> Sum45/1, Sum37/1
  Constant8/1 -> Sum40/2
  [Q4] -> Gain77/1
  [Vod2] -> Sum9/2
  Add20/1 -> Sum41/1
  Add9/1 -> Sum23/2
  Add18/1 -> Sum41/2
  Gain73/1 -> Add19/1
  Gain78/1 -> Add21/1
  [wo2] -> Sum26/1, Sum27/1, Sum28/1
  Switch/1 -> Add2/2
  Add22/1 -> Add23/1
  Gain25/1 -> Switch4/1
  Switch4/1 -> Add5/2
